simulink model "obstaculo2_quebra_mola_pibit_2025"  (R2025a)
settings: Solver=VariableStepAuto  StartTime=0.0  StopTime=10.0  RelTol=1e-3
values from neighbouring files (symbols this model uses):
  a_Ax = 0.070    (= 0.07)    [parametros_suspensao_completo_pibit_final.m]
  entre_eixos = 0.184356    [parametros_suspensao_completo_pibit_final.m]
  Hmax = 10/100    (= 0.1)    [parametros_suspensao_completo_pibit_final.m]
  Lqm = 3,7    [parametros_suspensao_completo_pibit_final.m]
  Vv = 5    [parametros_suspensao_completo_pibit_final.m]
undefined symbols (not defined in the file or in its folder): t_reto_diant, Xcg

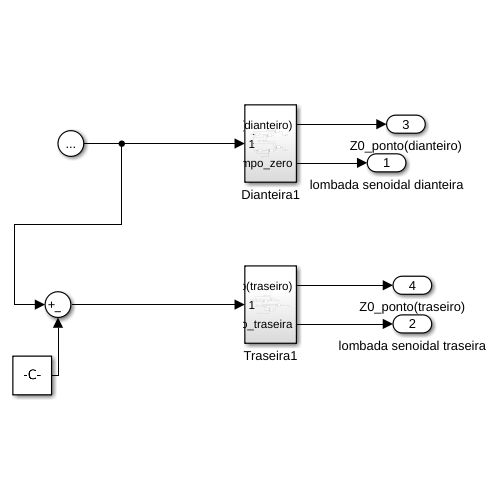
[thumbnail: Simulink's stored preview of the top-level diagram]
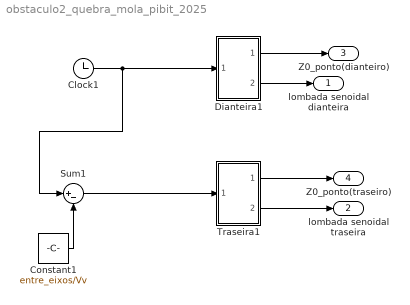
== system obstaculo2_quebra_mola_pibit_2025 ==
  Clock1 : Clock
  Constant1 : Constant  Value=entre_eixos/Vv
  Dianteira1 : Subsystem
  Sum1 : Sum  Inputs=|+-
  Traseira1 : Subsystem
  lombada senoidal dianteira : Outport
  lombada senoidal traseira : Outport  Port=2
  Z0_ponto(dianteiro) : Outport  Port=3
  Z0_ponto(traseiro) : Outport  Port=4
  wires:
  Clock1/1 -> Sum1/1, Dianteira1/1(In1)
  Traseira1/2(posicao_traseira) -> lombada senoidal traseira/1
  Sum1/1 -> Traseira1/1(In1)
  Dianteira1/2(posicao_desde_tempo_zero) -> lombada senoidal dianteira/1
  Constant1/1 -> Sum1/2
  Dianteira1/1(Z0_ponto(dianteiro)) -> Z0_ponto(dianteiro)/1
  Traseira1/1(Z0_ponto(traseiro)) -> Z0_ponto(traseiro)/1

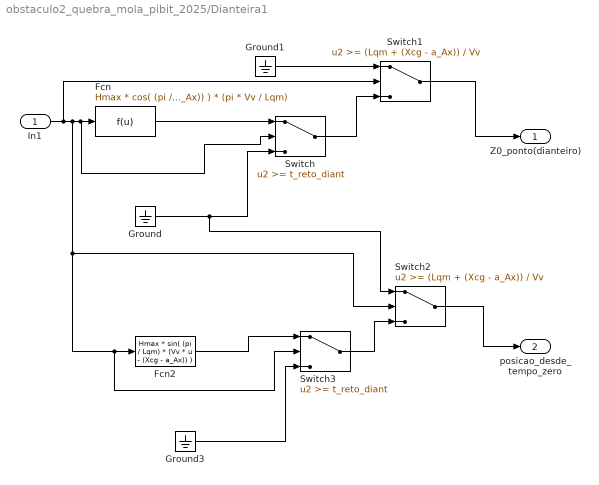
== system obstaculo2_quebra_mola_pibit_2025/Dianteira1 ==
  In1 : Inport
  Fcn : Fcn  Expr=Hmax * cos( (pi / Lqm) * (Vv * u - (Xcg - a_Ax)) ) * (pi * Vv / Lqm)
  Fcn2 : Fcn  Expr=Hmax * sin( (pi / Lqm) * (Vv * u - (Xcg - a_Ax)) )
  Ground : Ground
  Ground1 : Ground
  Ground3 : Ground
  Switch : Switch  Threshold=t_reto_diant  SaturateOnIntegerOverflow=off  InputSameDT=off
  Switch1 : Switch  Threshold=(Lqm + (Xcg - a_Ax)) / Vv  SaturateOnIntegerOverflow=off  InputSameDT=off
  Switch2 : Switch  Threshold=(Lqm + (Xcg - a_Ax)) / Vv  SaturateOnIntegerOverflow=off  InputSameDT=off
  Switch3 : Switch  Threshold=t_reto_diant  SaturateOnIntegerOverflow=off  InputSameDT=off
  Z0_ponto(dianteiro) : Outport
  posicao_desde_tempo_zero : Outport  Port=2
  wires:
  Switch/1 -> Switch1/3
  In1/1 -> Switch1/2, Switch2/2, Switch3/2, Fcn2/1, Fcn/1, Switch/2
  Fcn/1 -> Switch/1
  Ground1/1 -> Switch1/1
  Switch1/1 -> Z0_ponto(dianteiro)/1
  Ground/1 -> Switch2/1, Switch/3
  Switch2/1 -> posicao_desde_tempo_zero/1
  Fcn2/1 -> Switch3/1
  Switch3/1 -> Switch2/3
  Ground3/1 -> Switch3/3

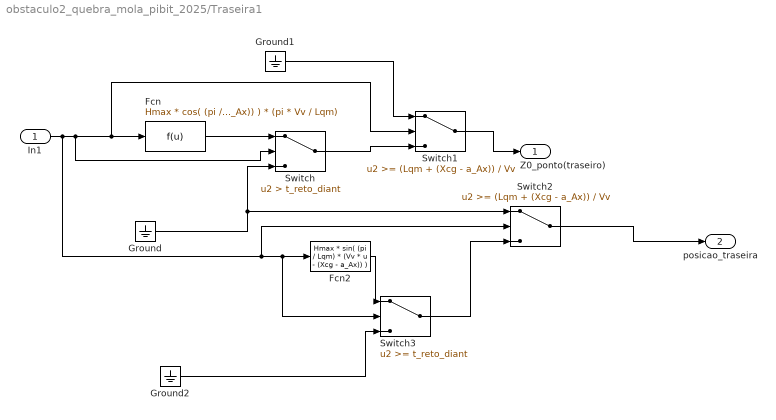
== system obstaculo2_quebra_mola_pibit_2025/Traseira1 ==
  In1 : Inport
  Fcn : Fcn  Expr=Hmax * cos( (pi / Lqm) * (Vv * u - (Xcg - a_Ax)) ) * (pi * Vv / Lqm)
  Fcn2 : Fcn  Expr=Hmax * sin( (pi / Lqm) * (Vv * u - (Xcg - a_Ax)) )
  Ground : Ground
  Ground1 : Ground
  Ground2 : Ground
  Switch : Switch  Criteria=u2 > Threshold  Threshold=t_reto_diant  SaturateOnIntegerOverflow=off  InputSameDT=off
  Switch1 : Switch  Threshold=(Lqm + (Xcg - a_Ax)) / Vv  SaturateOnIntegerOverflow=off  InputSameDT=off
  Switch2 : Switch  Threshold=(Lqm + (Xcg - a_Ax)) / Vv  SaturateOnIntegerOverflow=off  InputSameDT=off
  Switch3 : Switch  Threshold=t_reto_diant  SaturateOnIntegerOverflow=off  InputSameDT=off
  Z0_ponto(traseiro) : Outport
  posicao_traseira : Outport  Port=2
  wires:
  Ground/1 -> Switch/3, Switch2/1
  Fcn/1 -> Switch/1
  Ground1/1 -> Switch1/1
  Switch/1 -> Switch1/3
  Switch1/1 -> Z0_ponto(traseiro)/1
  Switch3/1 -> Switch2/3
  In1/1 -> Switch2/2, Switch3/2, Fcn2/1, Switch1/2, Fcn/1, Switch/2
  Fcn2/1 -> Switch3/1
  Switch2/1 -> posicao_traseira/1
  Ground2/1 -> Switch3/3
